simulink model "MPC"  (R2018a)
settings: Solver=VariableStepAuto  StartTime=0.0  StopTime=18  FixedStep=0.01  RelTol=1e-3
PreLoadFcn:
  | setUpPurePursuitCurveHighVel
model workspace (MAT data in the model file):
  firstWarning = 0
  originalScenarioChecksum = 'F73A6DA3C723D3CA73A6F931B7A52A9C'
values from neighbouring files (symbols this model uses):
  mu = m    [PSO_MPC.m]
  ref = i    [PSO_MPC.m]
  vx = j    [PSO_MPC.m]
  wy = l    [PSO_MPC.m]
undefined symbols (not defined in the file or in its folder): parms
libraries: autolibutils x4, autolibshared x3, vehdynlibviscommon x1, simulink x1
(part 3 of 3)

== matlab function MPC/MPC ==
  settings: updateMethod=DISCRETE
  data: u output; Vx input; u input; y input; r input; a input; N input; Nc input; Np input; R input; Qy input; u_min input; u_max input; deltau_min input; deltau_max input; y_min input; y_max input; xm input
function u = fcn(Vx, u,y,r,a,N,Nc,Np,R,Qy,u_min,u_max,deltau_min,deltau_max,y_min,y_max,xm)

tic;

coder.extrinsic('c2dm')
%coder.extrinsic(function)

%load('new_trajectory.mat')


% Model identification
persistent m,
if isempty(m)
  m = 1575;
end
persistent Iz,
if isempty(Iz)
  Iz = 2875;
end
persistent lr,
if isempty(lr)
  lr = 1.6;
end
persistent lf,
if isempty(lf)
  lf = 1.2;
end
persistent Cf,
if isempty(Cf)
  Cf = 19000;
end
persistent Cr,
if isempty(Cr)
  Cr = 33000;
end
persistent dt,
if isempty(dt)
  dt = 0.1;
end



%state vector  [y_dot phi phi_dot y]
Ac = [-(2*Cf+2*Cr)/m/Vx, 0, -Vx-(2*Cf*lf-2*Cr*lr)/m/Vx, 0;
     0, 0, 1, 0;
     -(2*Cf*lf-2*Cr*lr)/Iz/Vx, 0, -(2*Cf*lf^2+2*Cr*lr^2)/Iz/Vx, 0;
     1, Vx, 0, 0];
Bc = [2*Cf/m 0 2*Cf*lf/Iz 0]';   
Cc = [0 0 0 1];
%C2 = [0 0 0 1; 0 1 0 0];
Dc = zeros(1,1);


[Ad, Bd, Cd, Dd]=c2dm(Ac,Bc,Cc,Dc,dt,'zoh');
% tic
% Make the augmented state-space model
n1 = 0;
m1 = 0;
n_in = 0;

[m1, n1] = size(Cd);
[n1, n_in] = size(Bd);
A = eye(n1+m1, n1+m1);
A(1:n1, 1:n1) = Ad;
A(n1+1:n1+m1,1:n1) = Cd*Ad;
B = zeros(n1+m1, n_in);
B(1:n1,:) = Bd;
B(n1+1:n1+m1,:) = Cd*Bd;
C = zeros(m1, n1+m1);
C(:, n1+1:n1+m1) = eye(m1, m1);
D = Dd;


%obtain constraints data matrices

[M1,Lzerot]=Mdu(a,N,1,Nc);
M0=Mu(a,N,1,Nc);

%initial conditions for closed-loop simulation using constrained control
%specify the limits for ?u and u


persistent xm_old
if isempty(xm_old)
  %xm_old=[0; 0; 0; 37];
  xm_old=zeros(4,1);
end


persistent Xf
if isempty(Xf)
  Xf=[xm; y-r];
end


Xf=[xm-xm_old;y-r];
%end
xm_old=xm;


y_bar_min=y_min-r;
y_bar_max=y_max-r;


up=u;


Q=[0,0,0,0,0;0,0,0,0,0;0,0,0,0,0;0,0,0,0,0;0,0,0,0,Qy];



[Phi,F]=mpcgain(Ad,Bd,Cd,N,Np);
[Omega,Psi]=dmpc(A,B,a,N,Np,Q,R);







%% constrains on U first
 M=[M0;-M0;M1;-M1;Phi(1:Nc,1)*Lzerot;-Phi(1:Nc,1)*Lzerot];


%closed-loop simulation performed recursively
%optimal control is also found recursively

%% constrains on u first
gamma=[(u_max-up)*ones(Nc,1);(-u_min+up)*ones(Nc,1);...
    deltau_max*ones(Nc,1);-deltau_min*ones(Nc,1);...
    y_bar_max-F(1:Nc,:)*Xf;-y_bar_min+F(1:Nc,:)*Xf];

eta=QPhild(Omega,Psi*Xf,M,gamma);

deltau=Lzerot*eta;
if (deltau>deltau_max) deltau=deltau_max;end
if (deltau<deltau_min) deltau=deltau_min;end
u=u+deltau;
if (u>u_max) deltau=u_max-up; u=u_max; end
if (u<u_min) deltau=u_min-up; u=u_min; end
